simulink subsystem "distanceFromCenter"  (R2019b)
settings: Solver=VariableStepAuto  StartTime=0.0  StopTime=10.0  RelTol=1e-3
settings Model: Creator=maudvanlent  LastModifiedBy=maudvanlent

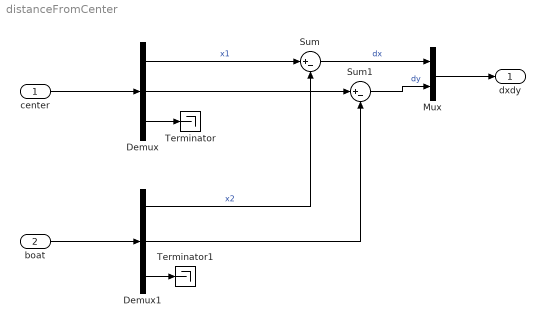
== system distanceFromCenter ==
  center : Inport
  boat : Inport  Port=2
  Demux : Demux  Outputs=3
  Demux1 : Demux  Outputs=3
  Mux : Mux  Inputs=2
  Sum : Sum  Inputs=|+-
  Sum1 : Sum  Inputs=|+-
  Terminator : Terminator
  Terminator1 : Terminator
  dxdy : Outport
  wires:
  Demux1/1 -> Sum/2  "x2"
  Demux/1 -> Sum/1  "x1"
  Mux/1 -> dxdy/1
  Sum/1 -> Mux/1  "dx"
  Demux/2 -> Sum1/1
  Sum1/1 -> Mux/2  "dy"
  Demux1/2 -> Sum1/2
  boat/1 -> Demux1/1
  Demux/3 -> Terminator/1
  Demux1/3 -> Terminator1/1
  center/1 -> Demux/1
